simulink model "trainn_traction_system_4motors_CRH3_ver1"  (R2020b)
settings: Solver=VariableStepAuto  StartTime=0.0  StopTime=3  RelTol=1e-3
model workspace (MAT data in the model file):
  C = 0.016
  J = 5
  L = 0.005
  Llr = 0.006
  Lls = 0.001416
  Lm = 0.0254
  R = 0.2
  Rr = 0.16
  Rs = 0.15
  T = 1e-06
  Tloadmax = 100
  Tloadstart = 2
  Tpwm = 0.0001
  Ts = 0.0008
  Vdc_ref = 2700
  Vpeak = 1550
  f = 50
  noiseDense = 0.01
  np = 2
  sample_time = 2e-05
  tE1 = 3.25
  tE1w = 10
  tE2 = 10
  tE2w = 10
  tE3 = 10
  tE3w = 10
  tE4 = 10
  tE4w = 10
  t_precharge = 0.15
  w = 314.159265359
libraries: powerlib x19, simulink x19, pid_lib x1, eeSinusoidalMeasurementV2 x1
(part 3 of 3)

== matlab function trainn_traction_system_4motors_CRH3_ver1/motor module4/电机控制模块/SVPWM/ Gen Gate ==
  data: t input; t0 input; Ts input; T0 input; T1 input; T2 input; sec input; g output
function g = fcn( t, t0,  Ts, T0, T1, T2, sec)
% T0 = params(1);
% T1 = params(2);
% T2 = params(3);
% sec = params(4);
dt = t - t0;



t_left1 = T0/4;
t_right1 = Ts - T0/4;

t_left2_odd_sec = t_left1 + T1/2;
t_left2_eve_sec = t_left1 + T2/2;
t_left3 = T0/4 + T1/2 + T2/2;
t_right3 = 3*T0/4 + T1/2 + T2/2;
t_right2_odd_sec = Ts - T0/4 - T1/2;
t_right2_eve_sec = Ts - T0/4 - T2/2;


gA = 0;
gB = 0;
gC = 0;

switch sec
    case 1
        if(dt >= t_left1 && dt <= t_right1)
            gA = 1;
        else
            gA = 0;
        end
        if(dt >= t_left2_odd_sec && dt <= t_right2_odd_sec)
            gB = 1;
        else
            gB = 0;
        end
        if(dt >= t_left3 && dt <= t_right3)
            gC = 1;
        else
            gC = 0;
        end
    case 2
        if(dt >= t_left1 && dt <= t_right1)
            gB = 1;
        else
            gB = 0;
        end
        if(dt >= t_left2_eve_sec && dt <= t_right2_eve_sec)
            gA = 1;
        else
            gA = 0;
        end
        if(dt >= t_left3 && dt <= t_right3)
            gC = 1;
        else
            gC = 0;
        end
    case 3
        if(dt >= t_left1 && dt <= t_right1)
            gB = 1;
        else
            gB = 0;
        end
        if(dt >= t_left2_odd_sec && dt <= t_right2_odd_sec)
            gC = 1;
        else
            gC = 0;
        end
        if(dt >= t_left3 && dt <= t_right3)
            gA = 1;
        else
            gA = 0;
        end
    case 4
        if(dt >= t_left1 && dt <= t_right1)
            gC = 1;
        else
            gC = 0;
        end
        if(dt >= t_left2_eve_sec && dt <= t_right2_eve_sec)
            gB = 1;
        else
            gB = 0;
        end
        if(dt >= t_left3 && dt <= t_right3)
            gA = 1;
        else
            gA = 0;
        end
    case 5
        if(dt >= t_left1 && dt <= t_right1)
            gC = 1;
        else
            gC = 0;
        end
        if(dt >= t_left2_odd_sec && dt <= t_right2_odd_sec)
            gA = 1;
        else
            gA = 0;
        end
        if(dt >= t_left3 && dt <= t_right3)
            gB = 1;
        else
            gB = 0;
        end
    case 6
        if(dt > t_left1 && dt < t_right1)
            gA = 1;
        else
            gA = 0;
        end
        if(dt > t_left2_eve_sec && dt < t_right2_eve_sec)
            gC = 1;
        else
            gC = 0;
        end
        if(dt > t_left3 && dt < t_right3)
            gB = 1;
        else
            gB = 0;
        end    
end
g = [gA; 1-gA; gB; 1-gB; gC; 1-gC];

== matlab function trainn_traction_system_4motors_CRH3_ver1/motor module4/电机控制模块/SVPWM/MATLAB Function1 ==
  data: old_t0 input; t input; trigger input; T0 input; new_t0 output; newT0 output; T1 input; T2 input; sec input; oldT0 input; oldT1 input; oldT2 input; oldSec input; newT1 output; newT2 output; newSec output
% function [new_t0, newT] = fcn( old_t0,  t, trigger, T, oldT)
function [new_t0, newT0, newT1, newT2, newSec] = fcn( old_t0,  t, trigger, T0, T1, T2, sec, oldT0, oldT1, oldT2, oldSec)
if(trigger)
    newT0 = T0;
    newT1 = T1;
    newT2 = T2;
    newSec = sec;
    new_t0 = t;
else
    new_t0 = old_t0;
    newT0 = oldT0;
    newT1 = oldT1;
    newT2 = oldT2;
    newSec = oldSec;
end

== matlab function trainn_traction_system_4motors_CRH3_ver1/motor module4/电机控制模块/SVPWM/MATLAB Function3 ==
  data: Udc input; T0 output; Ualpha input; Ubeta input; Ts input; sec input; T1 output; T2 output

function [T0, T1, T2] = fcn( Udc, Ualpha, Ubeta,  Ts, sec)
co = cos((sec-1)*pi/3);
si = sin((sec-1)*pi/3);

Ualpha_ = Ualpha*co + Ubeta*si;
Ubeta_ = -Ualpha*si + Ubeta*co;


T2 = sqrt(3)*Ubeta_/Udc*Ts;
T1 = ( 3*Ualpha_ - sqrt(3)* Ubeta_)/2/Udc*Ts;
T0 = Ts - T1 - T2;

== matlab function trainn_traction_system_4motors_CRH3_ver1/motor module1/Subsystem1/SVPWM1/MATLAB Function10 ==
  data: Ta input; gA output; Tb input; Tpwm input; section input; t input; gAN output; gB output; gBN output; gC output; gCN output
function [gA,gAN, gB, gBN, gC, gCN]  = fcn(Ta, Tb, Tpwm, section, t)

gA = (1==1);
gB = (1==1);
gC = (1==1);

T0 = Tpwm - Ta - Tb;

% 七段式 SPWM，扇区 1~6，对应6个扇区

if(mod(section, 2) == 1 ) % 1、3、5扇区
    t1 = T0/4;
    t2 = t1 + Ta / 2;
    t3 = t2 + Tb / 2;
    t4 = t3 + T0 / 2;
    t5 = t4 + Tb / 2;
    t6 = t5 + Ta / 2;
    
    if(section == 1)
        gA = (t >=t1 && t <=t6);
        gB = (t >=t2 && t <= t5);
        gC = (t >=t3 && t <= t4);
    elseif(section == 3)
        gB = (t >=t1 && t <=t6);
        gC = (t >=t2 && t <= t5);
        gA = (t >=t3 && t <= t4);
    else
        gC = (t >=t1 && t <=t6);
        gA = (t >=t2 && t <= t5);
        gB = (t >=t3 && t <= t4);
    end
else
    t1 = T0/4;
    t2 = t1 + Tb / 2;
    t3 = t2 + Ta / 2;
    t4 = t3 + T0 / 2;
    t5 = t4 + Ta / 2;
    t6 = t5 + Tb / 2;
    
    if(section == 2)
        gB = (t >=t1 && t <=t6);
        gA = (t >=t2 && t <= t5);
        gC = (t >=t3 && t <= t4);
    elseif(section == 4)
        gC = (t >=t1 && t <=t6);
        gB = (t >=t2 && t <= t5);
        gA = (t >=t3 && t <= t4);
    else
        gA = (t >=t1 && t <=t6);
        gC = (t >=t2 && t <= t5);
        gB = (t >=t3 && t <= t4);        
    end
    
end


gAN = ~gA;
gBN = ~gB;
gCN = ~gC;
% g = [gA, 1-gA, gB, 1-gB, gC, 1-gC];

== matlab function trainn_traction_system_4motors_CRH3_ver1/motor module4/电机控制模块/SVPWM/find section1/get section ==
  data: u input; y output
function y = fcn(u)
switch u
    case 5
        y = 1;
    case 7
        y = 2; 
    case 6
        y = 3;
    case 2
        y = 4;
    case 0
        y = 5;
    case 1
        y = 6;
    otherwise
        y = 0;
end

== matlab function trainn_traction_system_4motors_CRH3_ver1/motor module1/Subsystem1/SVPWM1/find section1/get section ==
  data: u input; y output
function y = fcn(u)
switch u
    case 5
        y = 1;
    case 7
        y = 2; 
    case 6
        y = 3;
    case 2
        y = 4;
    case 0
        y = 5;
    case 1
        y = 6;
    otherwise
        y = 0;
end

== matlab function trainn_traction_system_4motors_CRH3_ver1/motor module2/Subsystem2/SVPWM1/MATLAB Function10 ==
  data: Ta input; gA output; Tb input; Tpwm input; section input; t input; gAN output; gB output; gBN output; gC output; gCN output
function [gA,gAN, gB, gBN, gC, gCN]  = fcn(Ta, Tb, Tpwm, section, t)

gA = (1==1);
gB = (1==1);
gC = (1==1);

T0 = Tpwm - Ta - Tb;

% 七段式 SPWM，扇区 1~6，对应6个扇区

if(mod(section, 2) == 1 ) % 1、3、5扇区
    t1 = T0/4;
    t2 = t1 + Ta / 2;
    t3 = t2 + Tb / 2;
    t4 = t3 + T0 / 2;
    t5 = t4 + Tb / 2;
    t6 = t5 + Ta / 2;
    
    if(section == 1)
        gA = (t >=t1 && t <=t6);
        gB = (t >=t2 && t <= t5);
        gC = (t >=t3 && t <= t4);
    elseif(section == 3)
        gB = (t >=t1 && t <=t6);
        gC = (t >=t2 && t <= t5);
        gA = (t >=t3 && t <= t4);
    else
        gC = (t >=t1 && t <=t6);
        gA = (t >=t2 && t <= t5);
        gB = (t >=t3 && t <= t4);
    end
else
    t1 = T0/4;
    t2 = t1 + Tb / 2;
    t3 = t2 + Ta / 2;
    t4 = t3 + T0 / 2;
    t5 = t4 + Ta / 2;
    t6 = t5 + Tb / 2;
    
    if(section == 2)
        gB = (t >=t1 && t <=t6);
        gA = (t >=t2 && t <= t5);
        gC = (t >=t3 && t <= t4);
    elseif(section == 4)
        gC = (t >=t1 && t <=t6);
        gB = (t >=t2 && t <= t5);
        gA = (t >=t3 && t <= t4);
    else
        gA = (t >=t1 && t <=t6);
        gC = (t >=t2 && t <= t5);
        gB = (t >=t3 && t <= t4);        
    end
    
end


gAN = ~gA;
gBN = ~gB;
gCN = ~gC;
% g = [gA, 1-gA, gB, 1-gB, gC, 1-gC];

== matlab function trainn_traction_system_4motors_CRH3_ver1/motor module2/Subsystem2/SVPWM1/MATLAB Function3 ==
  data: Udc input; T0 output; Ualpha input; Ubeta input; Ts input; sec input; T1 output; T2 output

function [T0, T1, T2] = fcn( Udc, Ualpha, Ubeta,  Ts, sec)
co = cos((sec-1)*pi/3);
si = sin((sec-1)*pi/3);

Ualpha_ = Ualpha*co + Ubeta*si;
Ubeta_ = -Ualpha*si + Ubeta*co;


T2 = sqrt(3)*Ubeta_/Udc*Ts;
T1 = ( 3*Ualpha_ - sqrt(3)* Ubeta_)/2/Udc*Ts;
T0 = Ts - T1 - T2;

== matlab function trainn_traction_system_4motors_CRH3_ver1/motor module2/Subsystem2/SVPWM1/find section1/get section ==
  data: u input; y output
function y = fcn(u)
switch u
    case 5
        y = 1;
    case 7
        y = 2; 
    case 6
        y = 3;
    case 2
        y = 4;
    case 0
        y = 5;
    case 1
        y = 6;
    otherwise
        y = 0;
end

== matlab function trainn_traction_system_4motors_CRH3_ver1/motor module3/Subsystem3/SVPWM1/MATLAB Function10 ==
  data: Ta input; gA output; Tb input; Tpwm input; section input; t input; gAN output; gB output; gBN output; gC output; gCN output
function [gA,gAN, gB, gBN, gC, gCN]  = fcn(Ta, Tb, Tpwm, section, t)

gA = (1==1);
gB = (1==1);
gC = (1==1);

T0 = Tpwm - Ta - Tb;

% 七段式 SPWM，扇区 1~6，对应6个扇区

if(mod(section, 2) == 1 ) % 1、3、5扇区
    t1 = T0/4;
    t2 = t1 + Ta / 2;
    t3 = t2 + Tb / 2;
    t4 = t3 + T0 / 2;
    t5 = t4 + Tb / 2;
    t6 = t5 + Ta / 2;
    
    if(section == 1)
        gA = (t >=t1 && t <=t6);
        gB = (t >=t2 && t <= t5);
        gC = (t >=t3 && t <= t4);
    elseif(section == 3)
        gB = (t >=t1 && t <=t6);
        gC = (t >=t2 && t <= t5);
        gA = (t >=t3 && t <= t4);
    else
        gC = (t >=t1 && t <=t6);
        gA = (t >=t2 && t <= t5);
        gB = (t >=t3 && t <= t4);
    end
else
    t1 = T0/4;
    t2 = t1 + Tb / 2;
    t3 = t2 + Ta / 2;
    t4 = t3 + T0 / 2;
    t5 = t4 + Ta / 2;
    t6 = t5 + Tb / 2;
    
    if(section == 2)
        gB = (t >=t1 && t <=t6);
        gA = (t >=t2 && t <= t5);
        gC = (t >=t3 && t <= t4);
    elseif(section == 4)
        gC = (t >=t1 && t <=t6);
        gB = (t >=t2 && t <= t5);
        gA = (t >=t3 && t <= t4);
    else
        gA = (t >=t1 && t <=t6);
        gC = (t >=t2 && t <= t5);
        gB = (t >=t3 && t <= t4);        
    end
    
end


gAN = ~gA;
gBN = ~gB;
gCN = ~gC;
% g = [gA, 1-gA, gB, 1-gB, gC, 1-gC];

== matlab function trainn_traction_system_4motors_CRH3_ver1/motor module3/Subsystem3/SVPWM1/MATLAB Function3 ==
  data: Udc input; T0 output; Ualpha input; Ubeta input; Ts input; sec input; T1 output; T2 output

function [T0, T1, T2] = fcn( Udc, Ualpha, Ubeta,  Ts, sec)
co = cos((sec-1)*pi/3);
si = sin((sec-1)*pi/3);

Ualpha_ = Ualpha*co + Ubeta*si;
Ubeta_ = -Ualpha*si + Ubeta*co;


T2 = sqrt(3)*Ubeta_/Udc*Ts;
T1 = ( 3*Ualpha_ - sqrt(3)* Ubeta_)/2/Udc*Ts;
T0 = Ts - T1 - T2;

== matlab function trainn_traction_system_4motors_CRH3_ver1/motor module3/Subsystem3/SVPWM1/find section1/get section ==
  data: u input; y output
function y = fcn(u)
switch u
    case 5
        y = 1;
    case 7
        y = 2; 
    case 6
        y = 3;
    case 2
        y = 4;
    case 0
        y = 5;
    case 1
        y = 6;
    otherwise
        y = 0;
end

== matlab function trainn_traction_system_4motors_CRH3_ver1/motor module4/电机控制模块/SVPWM1/MATLAB Function10 ==
  data: Ta input; gA output; Tb input; Tpwm input; section input; t input; gAN output; gB output; gBN output; gC output; gCN output
function [gA,gAN, gB, gBN, gC, gCN]  = fcn(Ta, Tb, Tpwm, section, t)

gA = (1==1);
gB = (1==1);
gC = (1==1);

T0 = Tpwm - Ta - Tb;

% 七段式 SPWM，扇区 1~6，对应6个扇区

if(mod(section, 2) == 1 ) % 1、3、5扇区
    t1 = T0/4;
    t2 = t1 + Ta / 2;
    t3 = t2 + Tb / 2;
    t4 = t3 + T0 / 2;
    t5 = t4 + Tb / 2;
    t6 = t5 + Ta / 2;
    
    if(section == 1)
        gA = (t >=t1 && t <=t6);
        gB = (t >=t2 && t <= t5);
        gC = (t >=t3 && t <= t4);
    elseif(section == 3)
        gB = (t >=t1 && t <=t6);
        gC = (t >=t2 && t <= t5);
        gA = (t >=t3 && t <= t4);
    else
        gC = (t >=t1 && t <=t6);
        gA = (t >=t2 && t <= t5);
        gB = (t >=t3 && t <= t4);
    end
else
    t1 = T0/4;
    t2 = t1 + Tb / 2;
    t3 = t2 + Ta / 2;
    t4 = t3 + T0 / 2;
    t5 = t4 + Ta / 2;
    t6 = t5 + Tb / 2;
    
    if(section == 2)
        gB = (t >=t1 && t <=t6);
        gA = (t >=t2 && t <= t5);
        gC = (t >=t3 && t <= t4);
    elseif(section == 4)
        gC = (t >=t1 && t <=t6);
        gB = (t >=t2 && t <= t5);
        gA = (t >=t3 && t <= t4);
    else
        gA = (t >=t1 && t <=t6);
        gC = (t >=t2 && t <= t5);
        gB = (t >=t3 && t <= t4);        
    end
    
end


gAN = ~gA;
gBN = ~gB;
gCN = ~gC;
% g = [gA, 1-gA, gB, 1-gB, gC, 1-gC];

== matlab function trainn_traction_system_4motors_CRH3_ver1/motor module4/电机控制模块/SVPWM1/MATLAB Function3 ==
  data: Udc input; T0 output; Ualpha input; Ubeta input; Ts input; sec input; T1 output; T2 output

function [T0, T1, T2] = fcn( Udc, Ualpha, Ubeta,  Ts, sec)
co = cos((sec-1)*pi/3);
si = sin((sec-1)*pi/3);

Ualpha_ = Ualpha*co + Ubeta*si;
Ubeta_ = -Ualpha*si + Ubeta*co;


T2 = sqrt(3)*Ubeta_/Udc*Ts;
T1 = ( 3*Ualpha_ - sqrt(3)* Ubeta_)/2/Udc*Ts;
T0 = Ts - T1 - T2;

== matlab function trainn_traction_system_4motors_CRH3_ver1/motor module4/电机控制模块/SVPWM1/find section1/get section ==
  data: u input; y output
function y = fcn(u)
switch u
    case 5
        y = 1;
    case 7
        y = 2; 
    case 6
        y = 3;
    case 2
        y = 4;
    case 0
        y = 5;
    case 1
        y = 6;
    otherwise
        y = 0;
end

== matlab function trainn_traction_system_4motors_CRH3_ver1/motor module1/Subsystem1/SVPWM1/MATLAB Function3 ==
  data: Udc input; T0 output; Ualpha input; Ubeta input; Ts input; sec input; T1 output; T2 output

function [T0, T1, T2] = fcn( Udc, Ualpha, Ubeta,  Ts, sec)
co = cos((sec-1)*pi/3);
si = sin((sec-1)*pi/3);

Ualpha_ = Ualpha*co + Ubeta*si;
Ubeta_ = -Ualpha*si + Ubeta*co;


T2 = sqrt(3)*Ubeta_/Udc*Ts;
T1 = ( 3*Ualpha_ - sqrt(3)* Ubeta_)/2/Udc*Ts;
T0 = Ts - T1 - T2;

== matlab function trainn_traction_system_4motors_CRH3_ver1/motor module2/Subsystem2/SVPWM/ Gen Gate ==
  data: t input; t0 input; Ts input; T0 input; T1 input; T2 input; sec input; g output
function g = fcn( t, t0,  Ts, T0, T1, T2, sec)
% T0 = params(1);
% T1 = params(2);
% T2 = params(3);
% sec = params(4);
dt = t - t0;



t_left1 = T0/4;
t_right1 = Ts - T0/4;

t_left2_odd_sec = t_left1 + T1/2;
t_left2_eve_sec = t_left1 + T2/2;
t_left3 = T0/4 + T1/2 + T2/2;
t_right3 = 3*T0/4 + T1/2 + T2/2;
t_right2_odd_sec = Ts - T0/4 - T1/2;
t_right2_eve_sec = Ts - T0/4 - T2/2;


gA = 0;
gB = 0;
gC = 0;

switch sec
    case 1
        if(dt >= t_left1 && dt <= t_right1)
            gA = 1;
        else
            gA = 0;
        end
        if(dt >= t_left2_odd_sec && dt <= t_right2_odd_sec)
            gB = 1;
        else
            gB = 0;
        end
        if(dt >= t_left3 && dt <= t_right3)
            gC = 1;
        else
            gC = 0;
        end
    case 2
        if(dt >= t_left1 && dt <= t_right1)
            gB = 1;
        else
            gB = 0;
        end
        if(dt >= t_left2_eve_sec && dt <= t_right2_eve_sec)
            gA = 1;
        else
            gA = 0;
        end
        if(dt >= t_left3 && dt <= t_right3)
            gC = 1;
        else
            gC = 0;
        end
    case 3
        if(dt >= t_left1 && dt <= t_right1)
            gB = 1;
        else
            gB = 0;
        end
        if(dt >= t_left2_odd_sec && dt <= t_right2_odd_sec)
            gC = 1;
        else
            gC = 0;
        end
        if(dt >= t_left3 && dt <= t_right3)
            gA = 1;
        else
            gA = 0;
        end
    case 4
        if(dt >= t_left1 && dt <= t_right1)
            gC = 1;
        else
            gC = 0;
        end
        if(dt >= t_left2_eve_sec && dt <= t_right2_eve_sec)
            gB = 1;
        else
            gB = 0;
        end
        if(dt >= t_left3 && dt <= t_right3)
            gA = 1;
        else
            gA = 0;
        end
    case 5
        if(dt >= t_left1 && dt <= t_right1)
            gC = 1;
        else
            gC = 0;
        end
        if(dt >= t_left2_odd_sec && dt <= t_right2_odd_sec)
            gA = 1;
        else
            gA = 0;
        end
        if(dt >= t_left3 && dt <= t_right3)
            gB = 1;
        else
            gB = 0;
        end
    case 6
        if(dt > t_left1 && dt < t_right1)
            gA = 1;
        else
            gA = 0;
        end
        if(dt > t_left2_eve_sec && dt < t_right2_eve_sec)
            gC = 1;
        else
            gC = 0;
        end
        if(dt > t_left3 && dt < t_right3)
            gB = 1;
        else
            gB = 0;
        end    
end
g = [gA; 1-gA; gB; 1-gB; gC; 1-gC];

== matlab function trainn_traction_system_4motors_CRH3_ver1/motor module2/Subsystem2/SVPWM/MATLAB Function1 ==
  data: old_t0 input; t input; trigger input; T0 input; new_t0 output; newT0 output; T1 input; T2 input; sec input; oldT0 input; oldT1 input; oldT2 input; oldSec input; newT1 output; newT2 output; newSec output
% function [new_t0, newT] = fcn( old_t0,  t, trigger, T, oldT)
function [new_t0, newT0, newT1, newT2, newSec] = fcn( old_t0,  t, trigger, T0, T1, T2, sec, oldT0, oldT1, oldT2, oldSec)
if(trigger)
    newT0 = T0;
    newT1 = T1;
    newT2 = T2;
    newSec = sec;
    new_t0 = t;
else
    new_t0 = old_t0;
    newT0 = oldT0;
    newT1 = oldT1;
    newT2 = oldT2;
    newSec = oldSec;
end

== matlab function trainn_traction_system_4motors_CRH3_ver1/motor module2/Subsystem2/SVPWM/MATLAB Function3 ==
  data: Udc input; T0 output; Ualpha input; Ubeta input; Ts input; sec input; T1 output; T2 output

function [T0, T1, T2] = fcn( Udc, Ualpha, Ubeta,  Ts, sec)
co = cos((sec-1)*pi/3);
si = sin((sec-1)*pi/3);

Ualpha_ = Ualpha*co + Ubeta*si;
Ubeta_ = -Ualpha*si + Ubeta*co;


T2 = sqrt(3)*Ubeta_/Udc*Ts;
T1 = ( 3*Ualpha_ - sqrt(3)* Ubeta_)/2/Udc*Ts;
T0 = Ts - T1 - T2;
